simulink library "Problem_4"  (R2020a)
settings: Solver=VariableStepAuto  StartTime=0.0  StopTime=10.0  RelTol=1e-3
settings Model: Creator=Admin  LastModifiedBy=Admin

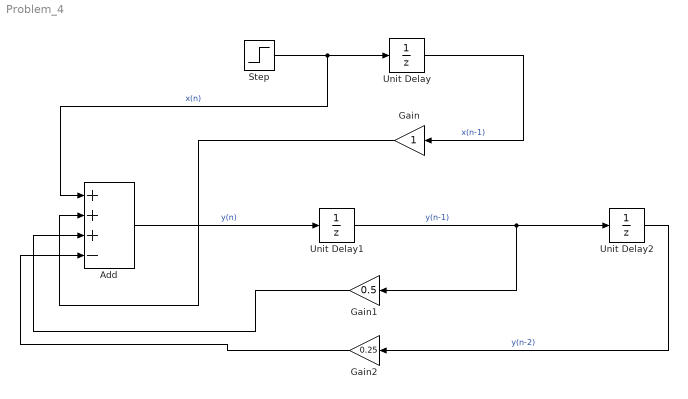
== system Problem_4 ==
  Add : Sum  Inputs=+++-
  Gain : Gain
  Gain1 : Gain  Gain=0.5
  Gain2 : Gain  Gain=0.25
  Step : Step  SampleTime=0
  Unit Delay : UnitDelay  SampleTime=-1  HasFrameUpgradeWarning=on
  Unit Delay1 : UnitDelay  SampleTime=-1  HasFrameUpgradeWarning=on
  Unit Delay2 : UnitDelay  SampleTime=-1  HasFrameUpgradeWarning=on
  wires:
  Unit Delay/1 -> Gain/1  "x(n-1)"
  Step/1 -> Add/1, Unit Delay/1  "x(n)"
  Unit Delay1/1 -> Unit Delay2/1, Gain1/1  "y(n-1)"
  Unit Delay2/1 -> Gain2/1  "y(n-2)"
  Gain2/1 -> Add/4
  Gain1/1 -> Add/3
  Gain/1 -> Add/2
  Add/1 -> Unit Delay1/1  "y(n)"
